simulink model "dspwwv"  (Simulink 8.3)
settings: Solver=FixedStepDiscrete  SolverMode=SingleTasking  StartTime=0.0  StopTime=inf  RelTol=1e-3  AbsTol=1e-6
model workspace (MATLAB code in the model file):
  | dlyVal = 2*rand(1);
libraries: simulink x5, dspsigops x2, dspmisc x1
Description:
  | WWV Digital Time-Code Receiver
CloseFcn:
  | clear ans;
settings Model: Creator=The MathWorks Inc.  ModifiedHistory=Initial Revision  CovMetricSettings=d  ExtModeTrigMode=oneshot  ExtModeArmWhenConnect=off  ExtModeAutoUpdateStatusClock=off
settings SolverCC: InsertRTBMode=Auto
settings DataIOCC: SaveOutput=off  SignalLogging=off  SaveTime=off  SignalLoggingName=sigsOut
settings OptimizationCC: InlineParams=on  InlineInvariantSignals=on  ExpressionDepthLimit=2147483647  RollThreshold=2  StateBitsets=on  DataBitsets=on  UseTempVars=on  InitFltsAndDblsToZero=on  EfficientFloat2IntCast=on  EfficientMapNaN2IntZero=off  AccelVerboseBuild=on
settings DebuggingCC: AlgebraicLoopMsg=error  SaveWithParameterizedLinksMsg=none  CheckExecutionContextPreStartOutputMsg=on  CheckExecutionContextRuntimeOutputMsg=on  SolverPrmCheckMsg=none  IntegerOverflowMsg=none  FcnCallInpInsideContextMsg=UseLocalSettings  UnconnectedOutputMsg=none
settings HardwareCC: ProdIntDivRoundTo=Zero  ProdHWDeviceType=Generic->Unspecified (assume 32-bit Generic)
settings SFSimCC: SFSimEcho=off  SimParseCustomCode=off
settings RTWCC: GenerateReport=on  RTWVerbose=off  LaunchReport=on  IncludeERTFirstTime=on
settings GRTTargetCC: TargetFcnLib=ansi_tfl_tmw.mat

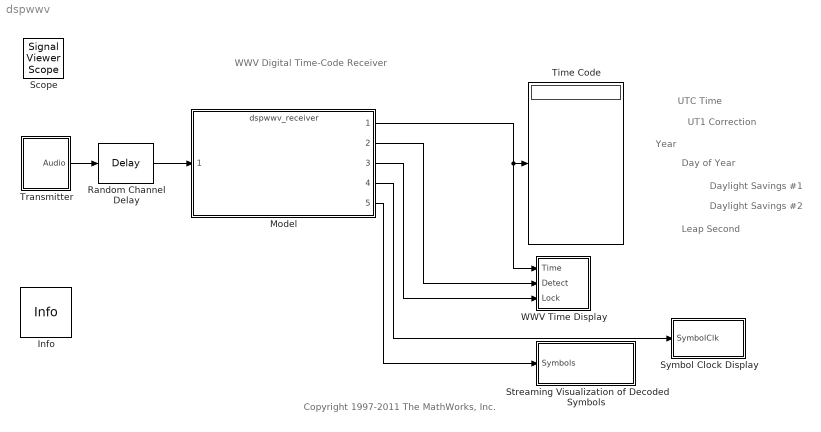
== system dspwwv ==
  note: UTC Time
  note: UT1 Correction
  note: Year
  note: Day of Year
  note: Daylight Savings #1
  note: Daylight Savings #2
  note: Leap Second
  note: WWV Digital Time-Code Receiver
  note: Copyright 1997-2011 The MathWorks, Inc.
  Info : dspmisc/Info  SystemSampleTime=-1
  Model : ModelReference  ModelNameDialog=dspwwv_receiver  SimulationMode=Normal  ModelReferenceVersion=1.113  CopyOfModelName=dspwwv_receiver  DefaultDataLogging=off
  Random Channel Delay : dspsigops/Delay  InputProcessing=Columns as channels (frame based)  dly_unit=Samples  delay=round(8000*dlyVal)  ic_detail=off  dif_ic_for_ch=off  dif_ic_for_dly=off  ic=0  reset_popup=None
  Streaming Visualization of Decoded Symbols : Subsystem  TreatAsAtomicUnit=on
      settings: RTWSystemCode=Nonreusable function
  Symbol Clock Display : Subsystem
  Time Code : Display
  Transmitter : Subsystem  TreatAsAtomicUnit=on  mask(IRIG-B Time Code Synthesizer){outp=Audio, dispTime=Current, utc=19.01, ut1=-0.3, day=201, yr=2006, dst=on, dst2=on, leap=off, bufsize=80}
      mask prompts: outp "Output:"; dispTime "Display time:"; utc "Time (hh.mm):"; ut1 "UT1 Correction ([-0.7, +0.7]):"; day "Day of year:"; yr "Year:"; dst "Daylight Savings"; dst2 "Daylight Savings #2"; leap "Leap second"; bufsize "Samples per frame:"
      mask help: Generate IRIG-B time code.
      mask init:
      | if strcmp(get_param(gcbh,'dispTime'),'Current')
      |     mode = 1;
      | else
      |     mode = 2;
      | end
      | 
      | x = [.1 .2 .2 .3 .3 .5 .5 .8 .8 .9];
      | y = [.2 .2 .8 .8 .2 .2 .8 .8 .2 .2];
      settings: RTWSystemCode=Nonreusable function
      mask Help: Generate IRIG-B time code.
      mask TypeOptions outp: Symbols | Audio
      mask TypeOptions dispTime: Current | User-specified
      mask Callback dispTime:
      | dTime = get_param(gcbh,'dispTime');
      | mask_visibles = get_param(gcbh,'MaskVisibilities');
      | if (strcmp(dTime,'User-specified'))
      |     for i = 3:9,
      |         mask_visibles{i} = 'on';
      |     end
      | else
      |     for i = 3:9,
      |         mask_visibles{i} = 'off';
      |     end
      | end
      | set_param(gcb,'MaskVisibilities',mask_visibles);
      | clear dTime mask_visibles i;
      mask Display: plot(x,y)
  WWV Time Display : Subsystem  TreatAsAtomicUnit=on  mask(WWV Time Display){FigPos=[670 475 230 230]}
      mask prompts: FigPos "Figure position:"
      mask help: Display WWV time-code data in a figure.
      settings: RTWSystemCode=Nonreusable function
      mask Help: Display WWV time-code data in a figure.
      mask Display: disp('WWV\nDisplay')
  Scope : SignalViewerScope  IOType=viewer  RefreshTime=0.035000
      settings: TimeRange=60
  wires:
  Transmitter/1(Audio) -> Random Channel Delay/1
  Model/1 -> Time Code/1, WWV Time Display/1(Time)
  Model/2 -> WWV Time Display/2(Detect)
  Model/3 -> WWV Time Display/3(Lock)
  Model/4 -> Symbol Clock Display/1(SymbolClk)
  Random Channel Delay/1 -> Model/1
  Model/5 -> Streaming Visualization of Decoded Symbols/1(Symbols)

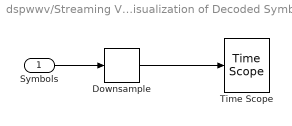
== system dspwwv/Streaming Visualization of Decoded Symbols ==
  Symbols : Inport
  Downsample : dspsigops/Downsample  N=80  phase=0  RateOptions=Allow multirate processing  smode=Allow multirate  fmode=Maintain input frame size  ic=0
  Time Scope : TimeScope  DefaultConfigurationName=spbscopes.TimeScopeBlockCfg  ScopeSpecification=DataTag2
  wires:
  Symbols/1 -> Downsample/1
  Downsample/1 -> Time Scope/1

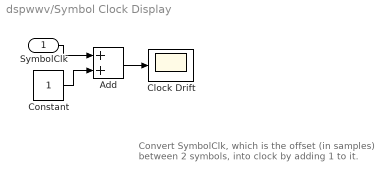
== system dspwwv/Symbol Clock Display ==
  note: Convert SymbolClk, which is the offset (in samples)
      | between 2 symbols, into clock by adding
      | 1 to it.
  SymbolClk : Inport
  Add : Sum
  Clock Drift : Scope
      settings: TimeRange=70  YMin=95  YMax=105  DataFormat=Structure
  Constant : Constant
  wires:
  Constant/1 -> Add/2
  Add/1 -> Clock Drift/1
  SymbolClk/1 -> Add/1

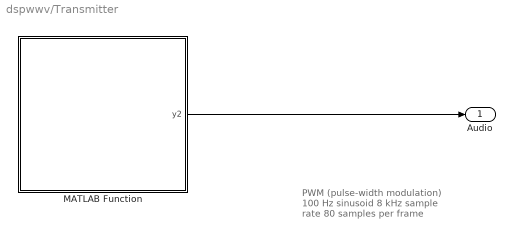
== system dspwwv/Transmitter ==
  note: PWM (pulse-width modulation)
      | 100 Hz sinusoid
      | 8 kHz sample rate
      | 80 samples per frame
  MATLAB Function : MATLAB Function  TreatAsAtomicUnit=on
  Audio : Outport
  wires:
  MATLAB Function/1(y2) -> Audio/1

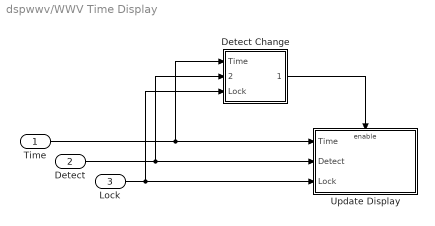
== system dspwwv/WWV Time Display ==
  Time : Inport
  Detect : Inport  Port=2
  Lock : Inport  Port=3
  Detect Change : Subsystem
  Update Display : Subsystem
  wires:
  Detect/1 -> Detect Change/2(Detect), Update Display/2(Detect)
  Lock/1 -> Detect Change/3(Lock), Update Display/3(Lock)
  Time/1 -> Detect Change/1(Time), Update Display/1(Time)
  Detect Change/1(Change) -> Update Display/Enable

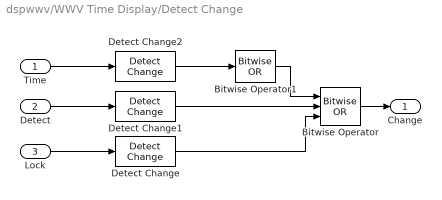
== system dspwwv/WWV Time Display/Detect Change ==
  Time : Inport
  Detect : Inport  Port=2
  Lock : Inport  Port=3
  Bitwise Operator : simulink/Logic and Bit Operations/Bitwise Operator  logicop=OR  UseBitMask=off  NumInputPorts=3  BitMask=bin2dec('11011001')  BitMaskRealWorld=Stored Integer
  Bitwise Operator1 : simulink/Logic and Bit Operations/Bitwise Operator  logicop=OR  UseBitMask=off  BitMask=bin2dec('11011001')  BitMaskRealWorld=Stored Integer
  Detect Change : simulink/Logic and Bit Operations/Detect Change  vinit=0  InputProcessing=Inherited  OutDataTypeStr=uint8
  Detect Change1 : simulink/Logic and Bit Operations/Detect Change  vinit=0  InputProcessing=Inherited  OutDataTypeStr=uint8
  Detect Change2 : simulink/Logic and Bit Operations/Detect Change  vinit=0  InputProcessing=Inherited  OutDataTypeStr=uint8
  Change : Outport
  wires:
  Detect Change2/1 -> Bitwise Operator1/1
  Detect Change1/1 -> Bitwise Operator/2
  Detect Change/1 -> Bitwise Operator/3
  Bitwise Operator1/1 -> Bitwise Operator/1
  Time/1 -> Detect Change2/1
  Detect/1 -> Detect Change1/1
  Lock/1 -> Detect Change/1
  Bitwise Operator/1 -> Change/1

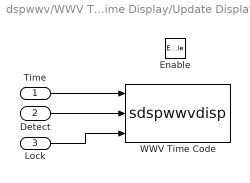
== system dspwwv/WWV Time Display/Update Display ==
  Time : Inport
  Detect : Inport  Port=2
  Lock : Inport  Port=3
  Enable : EnablePort
  WWV Time Code : M-S-Function  FunctionName=sdspwwvdisp  Parameters=FigPos
      settings: DeleteFcn=sdspwwvdisp('BlockDelete');  NameChangeFcn=sdspwwvdisp('NameChange');
  wires:
  Time/1 -> WWV Time Code/1
  Detect/1 -> WWV Time Code/2
  Lock/1 -> WWV Time Code/3

== matlab function Transmitter/MATLAB Function ==
  settings: updateMethod=DISCRETE  sampleTime=1/100
  data: y2 output double; mode parameter double; utc parameter double; ut1 parameter double; day parameter double; yr parameter double; dst parameter double; dst2 parameter double; leap parameter double
function y2 = gen_wwv_PWM_symbols(mode, utc, ut1, day, yr, dst, dst2, leap)
% This block supports the MATLAB subset.
% See the help menu for details. 

% Each symbol is represented with 8000 samples, that are transmitted at a
% rate of 80 samples/frame, and the frame period is 1/100 seconds. 
% This block outputs the Simulink frame of 80 samples every sample hit. 

persistent y1 idxSymbol idxSimFrame NumSimFramesPerSymbol ClockChangeSign

% Constants
PrePadOneSymbols = 5;
WWVSymbols = 60;
PostPadZeroSymbols = 3;
MaxSimFramesPerSymbol = 104;
MinSimFramesPerSymbol = 96;
NumSymbols = PrePadOneSymbols+WWVSymbols+PostPadZeroSymbols;


% Initialize persistent variables
% Initialize symbols vector
if isempty(y1), y1 = zeros(NumSymbols,1); end
% Initialize counter for symbols (goes from 1 to NumSymbols)
if isempty(idxSymbol), idxSymbol = 1; end
% Initialize counter for Simulation frame. For each symbol, the number of 
% simulation frames could be between MinSimFramesPerSymbol and MaxSimFramesPerSymbol. 
% Size of each frame is 80 samples. 
if isempty(idxSimFrame), idxSimFrame = 1; end
% Initialize number of simulation frames per symbol to MinSimFramesPerSymbol;
if isempty(NumSimFramesPerSymbol), NumSimFramesPerSymbol = MinSimFramesPerSymbol; end
% Initialize ClockChangeSign to gradually change NumSimFramesPerSymbol between 
% MinSimFramesPerSymbol and MaxSimFramesPerSymbol values
if isempty(ClockChangeSign), ClockChangeSign = 1; end

if (idxSymbol == 1) && (idxSimFrame == 1)
    % Compute the symbols only once per WWV Frame. 
    if (mode == 1),
        % Current mode
        x = getCurrentTimeStruct();
    else
        % User-specified mode, get the parameters from mask. 
        x = struct('yr',0,'leap',false,'utc',0,'ut1',0,'day',0,'dst',false,'dst2',false);
        x.utc     = utc;   % hh.mm
        x.ut1     = ut1;    % seconds in range [-0.7, +0.7]
        x.day     = day;     % day of year
        x.yr      = yr;    % year
        x.dst     = logical(dst);       % Daylight Savings Time indicator
        x.dst2    = logical(dst2);       % DST onset indicator
        x.leap    = logical(leap);       % Leap second    
    end

    % Generate symbol vector:
    y  = gen_irig(x);

    % Add a couple of symbols to the frame of data, so that
    % the decoder has time to synchronize:
    % Total number of symbols = 5+60+3 = 68.
    y1 = [ones(PrePadOneSymbols,1) ; y; zeros(PostPadZeroSymbols,1)]; 
end

% Generate modulated tone by doing Pulse width modulation on the WWV symbols.
% Generate NumSimFramesPerSymbol number of simulink frames for each symbol. 
y2 = single(zeros(80,1));
if (idxSimFrame <= NumSimFramesPerSymbol)
    y2 = gen_tone(y1(idxSymbol),idxSimFrame);
end

idxSimFrame = idxSimFrame+1;
if (idxSimFrame > NumSimFramesPerSymbol)
    % Keep looping the number of simulink frames per symbol between MinSimFramesPerSymbol and MaxSimFramesPerSymbol.
    NumSimFramesPerSymbol = NumSimFramesPerSymbol+ClockChangeSign*1;        
    if (NumSimFramesPerSymbol > MaxSimFramesPerSymbol),
        ClockChangeSign = -1;
        NumSimFramesPerSymbol = MaxSimFramesPerSymbol;
    end
    if (NumSimFramesPerSymbol < MinSimFramesPerSymbol),
        ClockChangeSign = 1;
        NumSimFramesPerSymbol = MinSimFramesPerSymbol;
    end
    idxSimFrame = 1;
    idxSymbol = idxSymbol+1;
    if (idxSymbol > NumSymbols)
        idxSymbol = 1;
    end
end

function s = gen_tone(x,whichSimFrame)
% Construct tone signal:
Ts = 1/8000;

%PMISS=0; 
P0   =1; 
P1   =2; 
PMARK=3; 

% Create (1/Ts) Hz sampled 100Hz PWM tone signal:
t  = 0:Ts:(0.01-Ts);
cs = single(cos(2*pi*100*t))';
s = single(zeros(80,1));
    
switch x
    case P0,
       if (whichSimFrame <= 17)
           s = cs;
       end
    case P1,
       if (whichSimFrame <= 47)
           s = cs;
       end
    case PMARK,
       if (whichSimFrame <= 77)
           s = cs;
       end
    otherwise,
end

return


% =======================

function y = gen_irig(x)

PMISS = 0;
P0    = 1;
%P1    = 2;
PMARK = 3;

% Preload with all P0's:
% ----------------------
y = P0*ones(60,1);

% 10-sec markers:
% ---------------
y(1:10:end) = PMARK;

% Start-of-frame marker:
% ----------------------
y(2) = PMISS;

% Data:
% -----
y(4)  = bit(x.dst2); % DST #2
y(57) = bit(x.dst);  % DST #1

y(5) = bit(x.leap);

ybcd = bcd(x.yr-1900,2);
y(6:9) = ybcd(1:4);
y(53:56) = ybcd(5:8);


hh = floor(x.utc);
mm = round((x.utc-hh)*100);
ybcd = bcd(mm,2);
y(12:15) = ybcd(1:4);
y(17:20) = ybcd(5:8);
ybcd = bcd(hh,2);
y(22:25) = ybcd(1:4);
y(27:30) = ybcd(5:8);

ybcda = bcd(x.day,3);
y(32:35) = ybcda(1:4);
y(37:40) = ybcda(5:8);
y(42:45) = ybcda(9:12);

y(52) = bit(sign(x.ut1)==-1);

ybcdb = bcd(abs(x.ut1*10),1);
y(58:60) = ybcdb(1:3);
return

% =======================

function y=bcd(d,n)
coder.extrinsic('find');
P0 = 1;
P1 = 2;
s=dec2bcd(d,n);
y=P0*ones(1,length(s)); % Set P0's
%y(find(s=='1'))=P1;    % Set P1's
for si = 1:length(s)
    if (s(si) == '1')
        y(si) = P1;
    end
end
y=fliplr(y);
return

% =======================

function y=bit(x)
P0    = 1;
P1    = 2;
if x, y=P1; else y=P0; end
return

% =======================

function y=dec2bcd(d,n)
%DEC2BCD Convert decimal integer to a binary-coded-decimal (BCD) string.
%   DEC2BCD(D) returns the BCD representation of D as a string.
%   D must be a non-negative integer.
%
%   DEC2BCD(D,N) produces a BCD representation with at least
%   N decimal digits encoded.
%
%   Example
%      dec2bcd(23) returns '00100011'
%      dec2bcd(23,3) returns '000000100011'
%
%   See also DEC2BIN, BIN2DEC, DEC2HEX, DEC2BASE.

coder.extrinsic('nargchk');
coder.extrinsic('error');
coder.extrinsic('dec2bin');

error(nargchk(1,2,nargin));

d = abs(d(:)); % Make sure d is a column vector.

digits = zeros(1,4);    
if d<2,
    numdigits=1;
else
    numdigits=ceil(log10(d));
end

if nargin>1,
	if (numel(n)~=1) || (numdigits<0),
	   error('N must be a positive scalar.');
    end
	n = round(n); % Make sure n is an integer.
else
  n = numdigits;
end

for i=numdigits-1:-1:0
  dig = floor(d*10^(-i));
  d = d - dig*(10^i);
  digits(4-i)=dig;
end

if (n == 1)
    digits1=digits(4);
    y=zeros(1,4);
elseif (n == 2)
    digits1=digits(3:4);    
    y=zeros(1,8);
elseif (n == 3) 
    digits1=digits(2:4);
    y=zeros(1,12);    
else
    digits1=digits;
    y=zeros(1,16);    
end

for i=1:length(digits1),
  if (i == 1)
    y(1:4)=dec2bin(digits1(i),4);
  elseif (i == 2)
    y(5:8)=dec2bin(digits1(i),4);
  elseif (i == 3)
    y(9:12)=dec2bin(digits1(i),4);
  else
    y(13:16)=dec2bin(digits1(i),4);
  end
end

%%%%%%%%%%%%%%%%%%%%%%%%%%%%%%%%%%%%%%%%%%%%%%%%%%%%%%%%%%%%%%%%%

function s = getCurrentTimeStruct()
coder.extrinsic('clock');
coder.extrinsic('num2str');
coder.extrinsic('str2double');
coder.extrinsic('warning');
time_vec = zeros(6,1);
time_vec = clock;
s = struct('yr',0,'leap',false,'utc',0,'ut1',0,'day',0,'dst',false,'dst2',false);
s.yr   = time_vec(1);
s.leap = (rem(time_vec(1),400)==0) || ((rem(time_vec(1),4)==0) && (rem(time_vec(1),100)~=0));

currentdateStr = num2str(time_vec(5));
if (isscalar(currentdateStr))
    s.utc=str2double([num2str(time_vec(4)) '.0' num2str(time_vec(5))]);
else
    s.utc=str2double([num2str(time_vec(4)) '.' num2str(time_vec(5))]);
end
s.ut1=-0.3;

ndays = getNumDaysForGivenDate(time_vec(2),time_vec(3),s.leap);

s.day=ndays;

s.dst=false;
s.dst2=false;

if (s.yr == 2008) 
    s.dst = isCurrentTimeDayLightSavings0(ndays,time_vec(4),3, 9, 11,2,s.leap);    
    s.dst2 = isCurrentTimeDayLightSavings0(ndays,time_vec(4),3,10, 11,3,s.leap);    
elseif (s.yr == 2009)
    s.dst = isCurrentTimeDayLightSavings0(ndays,time_vec(4),3, 8, 11,1,s.leap);    
    s.dst2 = isCurrentTimeDayLightSavings0(ndays,time_vec(4),3,9, 11,2,s.leap);    
elseif (s.yr == 2010)
    s.dst = isCurrentTimeDayLightSavings0(ndays,time_vec(4),3, 14, 11,7,s.leap);        
    s.dst2 = isCurrentTimeDayLightSavings0(ndays,time_vec(4),3, 15, 11,8,s.leap);        
elseif (s.yr == 2011)
    s.dst = isCurrentTimeDayLightSavings0(ndays,time_vec(4),3, 13, 11,6,s.leap);   
    s.dst2 = isCurrentTimeDayLightSavings0(ndays,time_vec(4),3,14, 11,7,s.leap);   
elseif (s.yr == 2012)
    s.dst = isCurrentTimeDayLightSavings0(ndays,time_vec(4),3, 11, 11,4,s.leap);   
    s.dst2 = isCurrentTimeDayLightSavings0(ndays,time_vec(4),3,12, 11,5,s.leap);   
elseif (s.yr == 2013)
    s.dst = isCurrentTimeDayLightSavings0(ndays,time_vec(4),3, 10, 11,3,s.leap);   
    s.dst2 = isCurrentTimeDayLightSavings0(ndays,time_vec(4),3,11, 11,4,s.leap);  
elseif (s.yr == 2014)
    s.dst = isCurrentTimeDayLightSavings0(ndays,time_vec(4),3, 9, 11,2,s.leap);   
    s.dst2 = isCurrentTimeDayLightSavings0(ndays,time_vec(4),3,10, 11,3,s.leap); 
elseif (s.yr == 2015)
    s.dst = isCurrentTimeDayLightSavings0(ndays,time_vec(4),3, 8, 11,1,s.leap);   
    s.dst2 = isCurrentTimeDayLightSavings0(ndays,time_vec(4),3,9, 11,2,s.leap);  
elseif (s.yr > 2015)
    warning('dspwwvgen:DSTWrong','Day light savings is not properly calculated');
end

% =======================
function ndays = getNumDaysForGivenDate(currMonth, currDay, isLeap)
if (isLeap)
    month_ndays = [31 29 31 30 31 30 31 31 30 31 30 31];
else
    month_ndays = [31 28 31 30 31 30 31 31 30 31 30 31];
end
ndays = 0;
for i = 1:(currMonth-1)
    ndays = ndays+month_ndays(i);
end
ndays = ndays + currDay;

% ===========================
function isDST = isCurrentTimeDayLightSavings0(currDay,currHour,startMonth, startDay, endMonth,endDay,isLeap)
isDST = false;
dayDSTStarts = getNumDaysForGivenDate(startMonth, startDay, isLeap);
datDSTEnds   = getNumDaysForGivenDate(endMonth, endDay, isLeap);
if (currDay >= dayDSTStarts) && (currDay <= datDSTEnds)
    if (currDay == dayDSTStarts)
        if (currHour >=2)
            isDST=true;
        end                
    elseif (currDay == datDSTEnds)
        if (currHour <=2)
            isDST=true;
        end                            
    else
        isDST=true;
    end
end
